simulink model "opg36"  (R2021b)
settings: Solver=FixedStepAuto  StartTime=0.9  StopTime=10  FixedStep=0.02  RelTol=1e-3
libraries: simulink x1
settings Model: Creator=klyx  LastModifiedBy=klyx

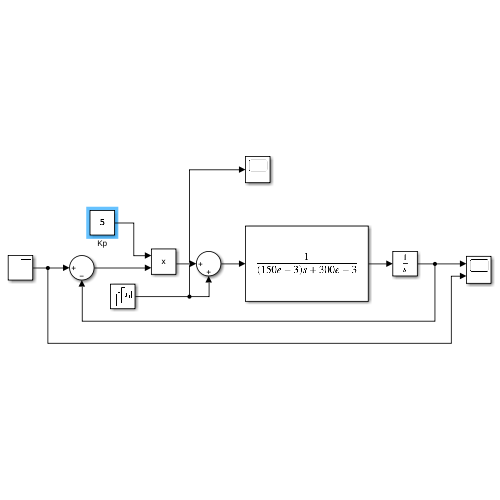
[thumbnail: Simulink's stored preview of the top-level diagram]
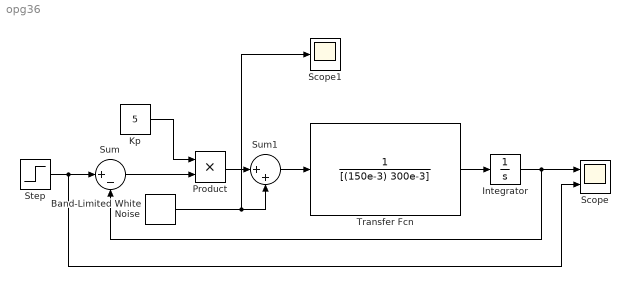
== system opg36 ==
  Band-Limited White Noise : simulink/Sources/Band-Limited White Noise  Cov=[0.1]  Ts=0.1  seed=[23341]
  Integrator : Integrator
  Kp : Constant  Value=5
  Product : Product
  Scope : Scope  NumInputPorts=2
  Scope1 : Scope
  Step : Step  SampleTime=0
  Sum : Sum  Inputs=|+-
  Sum1 : Sum  Inputs=|++
  Transfer Fcn : TransferFcn  Denominator=[(150e-3) 300e-3]
  wires:
  Step/1 -> Scope/2, Sum/1
  Sum/1 -> Product/2
  Kp/1 -> Product/1
  Transfer Fcn/1 -> Integrator/1
  Integrator/1 -> Sum/2, Scope/1
  Product/1 -> Sum1/1
  Sum1/1 -> Transfer Fcn/1
  Band-Limited White Noise/1 -> Sum1/2, Scope1/1
